simulink library "Lib_Solve_PWStateSpace_TMATS"  (R2015a)
settings: Solver=ode45  StartTime=0.0  StopTime=10.0  RelTol=1e-3
undefined symbols (not defined in the file): Atbl, Btbl, Ctbl, Dtbl, LinSys, Uo, Xo, Yo
Description:
  | Thomas Modules
settings Model: Creator=jwchapm2  LastModifiedBy=jwchapm2
settings OptimizationCC: ExpressionDepthLimit=2147483647
settings DebuggingCC: UnderspecifiedInitializationDetection=Classic  MergeDetectMultiDrivingBlocksExec=none  SolverPrmCheckMsg=warning  StateNameClashWarn=warning

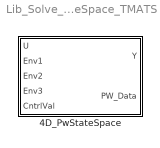
== system Lib_Solve_PWStateSpace_TMATS ==
  4D_PwStateSpace : Subsystem  mask(T-MATS: 4D Piecewise State Space Model Library Block){UisCntrl_M=off, NumEnv_M=three, XIC_M=[1 1], BN_M=double(gcb), ManDefLM_M=off, Env1_M=[0 0], Env2_M=[0 0], Env3_M=[0 0], CSVec_M=[0 0], Xsz_M=2, Ysz_M=3, Atbl_M=Atbl, Btbl_M=Btbl, Ctbl_M=Ctbl, Dtbl_M=Dtbl, Xo_M=Xo, Uo_M=Uo, Yo_M=Yo, SortEn_M=on, PLM_M=LinSys}
      mask prompts: UisCntrl_M "UisCntrl_M - Check if U is the control variable"; NumEnv_M "NumEnv_M - Number of Environmental variables"; XIC_M "XIC_M - X initial condition"; BN_M "BN_M - block name"; ManDefLM_M "ManDefLM_M - Manually define state-space model"; Env1_M "Env1_M - Environmental Vector 1 (m)"; Env2_M "Env2_M - Environmental Vector 2 (n)"; Env3_M "Env3_M - Environmental Vector 3 (p)"; CSVec_M "CSVec_M - Control Variable Vector (q)"; Xsz_M "Xnm_M - Number of states"; Ysz_M "Ynm_M - Number of outputs"; Atbl_M "Atbl_M - A matrix Array (mxnxpxqx(Xnm_M^2))"; Btbl_M "Btbl_M - B matrix Array (mxnxpxqx(Xnm_M))"; Ctbl_M "Ctbl_M - C matrix Array (mxnxpxqx(Xnm_M*Ynm_M))"; Dtbl_M "Dtbl_M - D matrix Array (mxnxpxqx(Ynm_M))"; Xo_M "Xo_M - X trim points (mxnxpxqx(Xnm_M))"; Uo_M "Uo_M - U trim points (mxnxpxq)"; Yo_M "Yo_M - Y trim points (mxnxpxqx(Ynm_M))"; SortEn_M "SortEn_M - Sort PW state-space model variables"; PLM_M "PLM_M - Piewise linear model structure name"
      mask help:
      | This block represents a 4D state-space model.
      |
      | This model will be of the form:
      | (xdot - xdot_0) = A*(x - x0) + B*(u - u0)
      | (y - y0) = C*(x - x0) + D*(u - u0)
      |
      | Where x is the system state, u is the system input (assumed to be 1x1), and y is the plant output.
      | 0 values are the trim point values.
      |
      | The 4 dimensions are represented as up to 3 "Environmental" parameters and 1 control parameter that may or may not be u. Note, if NumEnv_M is set to a value less than 3, tables must still be defined as 4D and unused Env values will be set to 0.
      mask init:
      | if NumEnv_M == 2
      |     if strcmp(get_param([BN_M '/Env2'],'BlockType'),'Constant')
      |         MSK_ReplaceBlock_TMATS([BN_M '/Env2'],'built-in/Inport');
      |     end
      |     if strcmp(get_param([BN_M '/Env3'],'BlockType'),'Inport')
      |         MSK_ReplaceBlock_TMATS([BN_M '/Env3'],'built-in/Constant');
      |         set_param([BN_M '/Env3'],'Value','[0]');
      |     end
      |     set_param([BN_M '/Env2'],'Port',num2str(3));
      | elseif NumEnv_M == 3
      |     if strcmp(get_param([BN_M '/Env2'],'BlockType'),'Constant')
      |         MSK_ReplaceBlock_TMATS([BN_M '/Env2'],'built-in/Inport');
      |     end
      |     set_param([BN_M '/Env2'],'Port',num2str(3));
      |     if strcmp(get_param([BN_M '/Env3'],'BlockType'),'Constant')
      |         MSK_ReplaceBlock_TMATS([BN_M '/Env3'],'built-in/Inport');
      |     end
      |     set_param([BN_M '/Env3'],'Port',num2str(4));
      | else
      |     if strcmp(get_param([BN_M '/Env2'],'BlockType'),'Inport')
      |         MSK_ReplaceBlock_TMATS([BN_M '/Env2'],'built-in/Constant');
      |         set_param([BN_M '/Env2'],'Value','[0]');
      |     end
      |     if strcmp(get_param([BN_M '/Env3'],'BlockType'),'Inport')
      |         MSK_ReplaceBlock_TMATS([BN_M '/Env3'],'built-in/Constant');
      |         set_param([BN_M '/Env3'],'Value','[0]');
      |     end
      | end
      | 
      | if UisCntrl_M == 0
      |     if strcmp(get_param([BN_M '/CntrlVal'],'BlockType'),'Constant')
      |         MSK_ReplaceBlock_TMATS([BN_M '/CntrlVal'],'built-in/Inport');
      |     end
      |     if NumEnv_M == 2
      |         set_param([BN_M '/CntrlVal'],'Port',num2str(4));
      |     elseif NumEnv_M == 3
      |         set_param([BN_M '/CntrlVal'],'Port',num2str(5));
      |     else
      |         set_param([BN_M '/CntrlVal'],'Port',num2str(3));
      |     end
      | elseif UisCntrl_M == 1
      |     if strcmp(get_param([BN_M '/CntrlVal'],'BlockType'),'Inport')
      |         MSK_ReplaceBlock_TMATS([BN_M '/CntrlVal'],'built-in/Constant');
      |         set_param([BN_M '/CntrlVal'],'Value','[0]');
      |     end
      | end
      | 
      | if ManDefLM_M
      |     %Manually define Linear model structure
      |     %Input axis vectors 4d
      |     PLM_M.EVec{1} = Env1_M;
      |     PLM_M.EVec{2} = Env2_M;
      |     PLM_M.EVec{3} = Env3_M;
      |     PLM_M.CSVec  = CSVec_M;
      |     %matrix sizes
      |     PLM_M.Asize = [Xsz_M Xsz_M];
      |     PLM_M.Bsize = [Xsz_M 1];
      |     PLM_M.Csize = [Ysz_M Xsz_M];
      |     PLM_M.Dsize = [Ysz_M 1];
      |     PLM_M.Xosize = [Xsz_M 1];
      |     PLM_M.Yosize = [Ysz_M 1];
      |     PLM_M.Uosize = 1;
      |     
      |     %define 5d tables (4d lookup, extra d relates different matrix
      |     %elements, ie. A11, A12,A21, A22.
      |     PLM_M.AtblFE = Atbl_M;
      |     PLM_M.BtblFE = Btbl_M;
      |     PLM_M.CtblFE = Ctbl_M;
      |     PLM_M.DtblFE = Dtbl_M;
      |     
      |     PLM_M.XoFE = Xo_M;
      |     PLM_M.UoFE = Uo_M;
      |     PLM_M.YoFE = Yo_M;
      | else
      |     % use structure linear system input... sort if necessary
      |     LS = PLM_M;
      |     
      |     if isfield(LS,'TblGen')
      |         if LS.TblGen == true;
      |             SortData = false;
      |         else
      |             SortData = true;
      |         end
      |     elseif all(isfield(LS,{'ABCD','EnvVec','X','U','Y','CntrlSlew'}))
      |         SortData = true;
      |     else
      |         SortData = false;
      |         sprintf(strcat('Warning in block: ',BN_M, ' Can not Sort out Linear system data due to improper PLM_M structure definition'))
      |     end
      |     
      |     if SortData == true && SortEn_M
      |         LS = TMATS_PWSort(LS);
      |         assignin('base','LinSys_Sorted',LS);
      |         PLM_M = LS;
      |     end
      | end
      mask Help: web(which('Solver_TMATS_PWSS.html'),'-helpbrowser')
      mask TypeOptions NumEnv_M: one | two | three
      mask Callback ManDefLM_M:
      | MSK_SEC_Enables_TMATS('ManDefLM_M',[6:18],'en')
      | MSK_SEC_Enables_TMATS('ManDefLM_M',[20],'dis')
      mask DialogControl Control2 Prompt: This tab is used when the state space model is defined using a structure.  (see block help)
      mask DialogControl Control2_copy Prompt: If this structure was generated using the T-MATS PW linear model generator, SortEn_M should be checked.

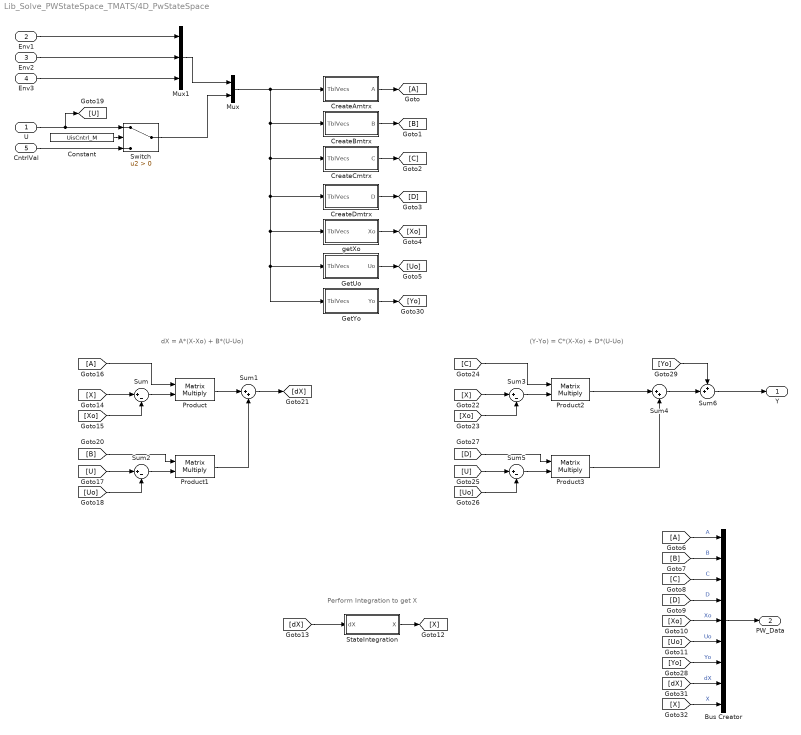
== system Lib_Solve_PWStateSpace_TMATS/4D_PwStateSpace ==
  note: dX = A*(X-Xo) + B*(U-Uo)
  note: Perform Integration to get X
  note: (Y-Yo) = C*(X-Xo) + D*(U-Uo)
  U : Inport
  Env1 : Inport  Port=2
  Env2 : Inport  Port=3
  Env3 : Inport  Port=4
  CntrlVal : Inport  Port=5
  Bus Creator : BusCreator  Inputs=9
  Constant : Constant  Value=UisCntrl_M
  CreateAmtrx : Subsystem
  CreateBmtrx : Subsystem
  CreateCmtrx : Subsystem
  CreateDmtrx : Subsystem
  GetUo : Subsystem
  GetYo : Subsystem
  Mux : Mux  Inputs=[3 1]
  Mux1 : Mux  Inputs=3
  Product{,1..3} (4 alike) : Product  Multiplication=Matrix(*)
  StateIntegration : Subsystem
  Sum{,2..3,5} (4 alike) : Sum  Inputs=|+-
  Sum1 : Sum  Inputs=|++
  Sum4 : Sum  Inputs=|++
  Sum6 : Sum  Inputs=++|
  Switch : Switch  Criteria=u2 > Threshold
  getXo : Subsystem
  Y : Outport
  PW_Data : Outport  Port=2
  wires:
  [X] -> Bus Creator/9  "X"
  [dX] -> Bus Creator/8  "dX"
  GetYo/1(Yo) -> [Yo]
  [Xo] -> Bus Creator/5  "Xo"
  [D] -> Bus Creator/4  "D"
  [C] -> Bus Creator/3  "C"
  [Uo] -> Bus Creator/6  "Uo"
  [B] -> Bus Creator/2  "B"
  [A] -> Bus Creator/1  "A"
  GetUo/1(Uo) -> [Uo]
  getXo/1(Xo) -> [Xo]
  U/1 -> [U], Switch/1
  CreateBmtrx/1(B) -> [B]
  CreateCmtrx/1(C) -> [C]
  CreateDmtrx/1(D) -> [D]
  Bus Creator/1 -> PW_Data/1
  [X] -> Sum/1
  [Xo] -> Sum/2
  Sum/1 -> Product/2
  [A] -> Product/1
  Product/1 -> Sum1/1
  [U] -> Sum2/1
  [Uo] -> Sum2/2
  Sum2/1 -> Product1/2
  [B] -> Product1/1
  Product1/1 -> Sum1/2
  Sum1/1 -> [dX]
  [X] -> Sum3/1
  [Xo] -> Sum3/2
  Sum3/1 -> Product2/2
  [C] -> Product2/1
  Product2/1 -> Sum4/1
  [U] -> Sum5/1
  [Uo] -> Sum5/2
  Sum5/1 -> Product3/2
  [D] -> Product3/1
  Product3/1 -> Sum4/2
  Sum6/1 -> Y/1
  Sum4/1 -> Sum6/2
  [Yo] -> Sum6/1
  [Yo] -> Bus Creator/7  "Yo"
  Env1/1 -> Mux1/1
  Constant/1 -> Switch/2
  CntrlVal/1 -> Switch/3
  CreateAmtrx/1(A) -> [A]
  Mux1/1 -> Mux/1
  Switch/1 -> Mux/2
  Mux/1 -> CreateBmtrx/1(TblVecs), CreateCmtrx/1(TblVecs), CreateDmtrx/1(TblVecs), getXo/1(TblVecs), GetUo/1(TblVecs), GetYo/1(TblVecs), CreateAmtrx/1(TblVecs)
  [dX] -> StateIntegration/1(dX)
  StateIntegration/1(X) -> [X]
  Env2/1 -> Mux1/2
  Env3/1 -> Mux1/3

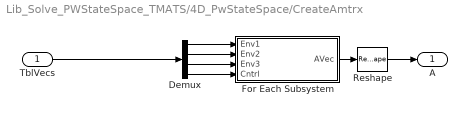
== system Lib_Solve_PWStateSpace_TMATS/4D_PwStateSpace/CreateAmtrx ==
  TblVecs : Inport
  Demux : Demux
  For Each Subsystem : Subsystem  TreatAsAtomicUnit=on  mask{Table=PLM_M.AtblFE}
  Reshape : Reshape  OutputDimensionality=Customize  OutputDimensions=PLM_M.Asize
  A : Outport
  wires:
  TblVecs/1 -> Demux/1
  Demux/2 -> For Each Subsystem/2(Env2)
  Reshape/1 -> A/1
  For Each Subsystem/1(AVec) -> Reshape/1
  Demux/3 -> For Each Subsystem/3(Env3)
  Demux/1 -> For Each Subsystem/1(Env1)
  Demux/4 -> For Each Subsystem/4(Cntrl)

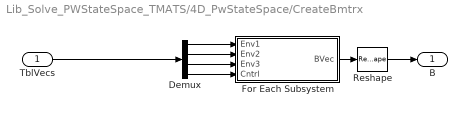
== system Lib_Solve_PWStateSpace_TMATS/4D_PwStateSpace/CreateBmtrx ==
  TblVecs : Inport
  Demux : Demux
  For Each Subsystem : Subsystem  TreatAsAtomicUnit=on  mask{Table=PLM_M.BtblFE}
  Reshape : Reshape  OutputDimensionality=Customize  OutputDimensions=PLM_M.Bsize
  B : Outport
  wires:
  Demux/4 -> For Each Subsystem/4(Cntrl)
  Demux/1 -> For Each Subsystem/1(Env1)
  Demux/3 -> For Each Subsystem/3(Env3)
  For Each Subsystem/1(BVec) -> Reshape/1
  Reshape/1 -> B/1
  Demux/2 -> For Each Subsystem/2(Env2)
  TblVecs/1 -> Demux/1

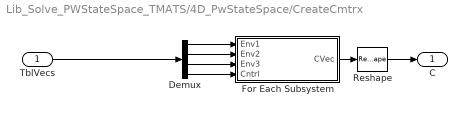
== system Lib_Solve_PWStateSpace_TMATS/4D_PwStateSpace/CreateCmtrx ==
  TblVecs : Inport
  Demux : Demux
  For Each Subsystem : Subsystem  TreatAsAtomicUnit=on  mask{Table=PLM_M.CtblFE}
  Reshape : Reshape  OutputDimensionality=Customize  OutputDimensions=PLM_M.Csize
  C : Outport
  wires:
  TblVecs/1 -> Demux/1
  Demux/2 -> For Each Subsystem/2(Env2)
  Reshape/1 -> C/1
  For Each Subsystem/1(CVec) -> Reshape/1
  Demux/3 -> For Each Subsystem/3(Env3)
  Demux/1 -> For Each Subsystem/1(Env1)
  Demux/4 -> For Each Subsystem/4(Cntrl)

== system Lib_Solve_PWStateSpace_TMATS/4D_PwStateSpace/CreateDmtrx ==
  TblVecs : Inport
  Demux : Demux
  For Each Subsystem : Subsystem  TreatAsAtomicUnit=on  mask{Table=PLM_M.DtblFE}
  Reshape : Reshape  OutputDimensionality=Customize  OutputDimensions=PLM_M.Dsize
  D : Outport
  wires:
  Demux/4 -> For Each Subsystem/4(Cntrl)
  Demux/1 -> For Each Subsystem/1(Env1)
  Demux/3 -> For Each Subsystem/3(Env3)
  For Each Subsystem/1(DVec) -> Reshape/1
  Reshape/1 -> D/1
  Demux/2 -> For Each Subsystem/2(Env2)
  TblVecs/1 -> Demux/1

== system Lib_Solve_PWStateSpace_TMATS/4D_PwStateSpace/GetUo ==
  TblVecs : Inport
  Demux : Demux
  Table lookup : Subsystem  TreatAsAtomicUnit=on  mask{Table=PLM_M.UoFE}
  Uo : Outport
  wires:
  Demux/4 -> Table lookup/4(Cntrl)
  Demux/1 -> Table lookup/1(Env1)
  Demux/3 -> Table lookup/3(Env3)
  Table lookup/1(UoVec) -> Uo/1
  Demux/2 -> Table lookup/2(Env2)
  TblVecs/1 -> Demux/1

== system Lib_Solve_PWStateSpace_TMATS/4D_PwStateSpace/GetYo ==
  TblVecs : Inport
  Demux : Demux
  For Each Subsystem : Subsystem  TreatAsAtomicUnit=on  mask{Table=PLM_M.YoFE}
  Reshape : Reshape  OutputDimensionality=Customize  OutputDimensions=PLM_M.Yosize
  Yo : Outport
  wires:
  Demux/4 -> For Each Subsystem/4(Cntrl)
  Demux/1 -> For Each Subsystem/1(Env1)
  Demux/3 -> For Each Subsystem/3(Env3)
  For Each Subsystem/1(YoVec) -> Reshape/1
  Reshape/1 -> Yo/1
  Demux/2 -> For Each Subsystem/2(Env2)
  TblVecs/1 -> Demux/1

== system Lib_Solve_PWStateSpace_TMATS/4D_PwStateSpace/StateIntegration ==
  dX : Inport  PortDimensions=length(XIC_M)
  Integrator : Integrator  InitialCondition=XIC_M
  X : Outport  PortDimensions=length(XIC_M)
  wires:
  Integrator/1 -> X/1
  dX/1 -> Integrator/1

== system Lib_Solve_PWStateSpace_TMATS/4D_PwStateSpace/getXo ==
  TblVecs : Inport
  Demux : Demux
  For Each Subsystem : Subsystem  TreatAsAtomicUnit=on  mask{Table=PLM_M.XoFE}
  Reshape : Reshape  OutputDimensionality=Customize  OutputDimensions=PLM_M.Xosize
  Xo : Outport
  wires:
  TblVecs/1 -> Demux/1
  Demux/2 -> For Each Subsystem/2(Env2)
  Reshape/1 -> Xo/1
  For Each Subsystem/1(XoVec) -> Reshape/1
  Demux/3 -> For Each Subsystem/3(Env3)
  Demux/1 -> For Each Subsystem/1(Env1)
  Demux/4 -> For Each Subsystem/4(Cntrl)

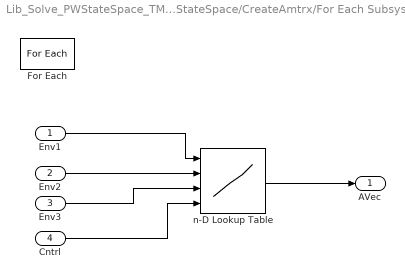
== system Lib_Solve_PWStateSpace_TMATS/4D_PwStateSpace/CreateAmtrx/For Each Subsystem ==
  Env1 : Inport  Partition=off
  Env2 : Inport  Port=2  Partition=off
  Env3 : Inport  Port=3  Partition=off
  Cntrl : Inport  Port=4  Partition=off
  For Each : ForEach  DisableCoverage=on  IterateSubsysMaskParameter=on  SubsysMaskParameterIterationDimension=5  IndexMode=One-based
  n-D Lookup Table : Lookup_n-D  NumberOfTableDimensions=4  BreakpointsForDimension1=PLM_M.EVec{1}  BreakpointsForDimension2=PLM_M.EVec{2}  BreakpointsForDimension3=PLM_M.EVec{3}  BreakpointsForDimension4=PLM_M.CSVec  Table=Table  InternalRulePriority=Speed  RndMeth=Simplest  InputSameDT=on
  AVec : Outport  ConcatenationDimension=1
  wires:
  n-D Lookup Table/1 -> AVec/1
  Cntrl/1 -> n-D Lookup Table/4
  Env3/1 -> n-D Lookup Table/3
  Env2/1 -> n-D Lookup Table/2
  Env1/1 -> n-D Lookup Table/1

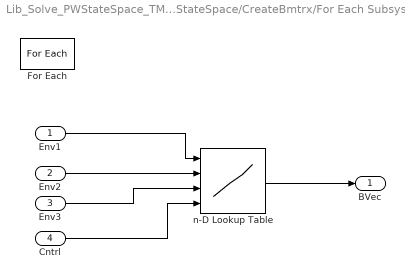
== system Lib_Solve_PWStateSpace_TMATS/4D_PwStateSpace/CreateBmtrx/For Each Subsystem ==
  Env1 : Inport  Partition=off
  Env2 : Inport  Port=2  Partition=off
  Env3 : Inport  Port=3  Partition=off
  Cntrl : Inport  Port=4  Partition=off
  For Each : ForEach  DisableCoverage=on  IterateSubsysMaskParameter=on  SubsysMaskParameterIterationDimension=5  IndexMode=One-based
  n-D Lookup Table : Lookup_n-D  NumberOfTableDimensions=4  BreakpointsForDimension1=PLM_M.EVec{1}  BreakpointsForDimension2=PLM_M.EVec{2}  BreakpointsForDimension3=PLM_M.EVec{3}  BreakpointsForDimension4=PLM_M.CSVec  Table=Table  InternalRulePriority=Speed  RndMeth=Simplest  InputSameDT=on
  BVec : Outport  ConcatenationDimension=1
  wires:
  Env1/1 -> n-D Lookup Table/1
  Env2/1 -> n-D Lookup Table/2
  Env3/1 -> n-D Lookup Table/3
  Cntrl/1 -> n-D Lookup Table/4
  n-D Lookup Table/1 -> BVec/1

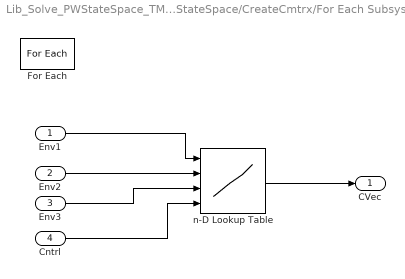
== system Lib_Solve_PWStateSpace_TMATS/4D_PwStateSpace/CreateCmtrx/For Each Subsystem ==
  Env1 : Inport  Partition=off
  Env2 : Inport  Port=2  Partition=off
  Env3 : Inport  Port=3  Partition=off
  Cntrl : Inport  Port=4  Partition=off
  For Each : ForEach  DisableCoverage=on  IterateSubsysMaskParameter=on  SubsysMaskParameterIterationDimension=5  IndexMode=One-based
  n-D Lookup Table : Lookup_n-D  NumberOfTableDimensions=4  BreakpointsForDimension1=PLM_M.EVec{1}  BreakpointsForDimension2=PLM_M.EVec{2}  BreakpointsForDimension3=PLM_M.EVec{3}  BreakpointsForDimension4=PLM_M.CSVec  Table=Table  InternalRulePriority=Speed  RndMeth=Simplest  InputSameDT=on
  CVec : Outport  ConcatenationDimension=1
  wires:
  n-D Lookup Table/1 -> CVec/1
  Cntrl/1 -> n-D Lookup Table/4
  Env3/1 -> n-D Lookup Table/3
  Env2/1 -> n-D Lookup Table/2
  Env1/1 -> n-D Lookup Table/1

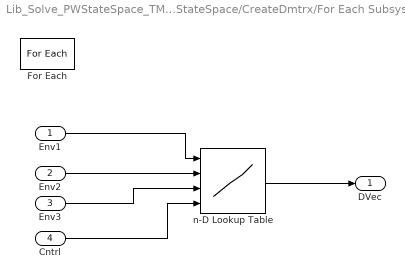
== system Lib_Solve_PWStateSpace_TMATS/4D_PwStateSpace/CreateDmtrx/For Each Subsystem ==
  Env1 : Inport  Partition=off
  Env2 : Inport  Port=2  Partition=off
  Env3 : Inport  Port=3  Partition=off
  Cntrl : Inport  Port=4  Partition=off
  For Each : ForEach  DisableCoverage=on  IterateSubsysMaskParameter=on  SubsysMaskParameterIterationDimension=5  IndexMode=One-based
  n-D Lookup Table : Lookup_n-D  NumberOfTableDimensions=4  BreakpointsForDimension1=PLM_M.EVec{1}  BreakpointsForDimension2=PLM_M.EVec{2}  BreakpointsForDimension3=PLM_M.EVec{3}  BreakpointsForDimension4=PLM_M.CSVec  Table=Table  InternalRulePriority=Speed  RndMeth=Simplest  InputSameDT=on
  DVec : Outport  ConcatenationDimension=1
  wires:
  Env1/1 -> n-D Lookup Table/1
  Env2/1 -> n-D Lookup Table/2
  Env3/1 -> n-D Lookup Table/3
  Cntrl/1 -> n-D Lookup Table/4
  n-D Lookup Table/1 -> DVec/1

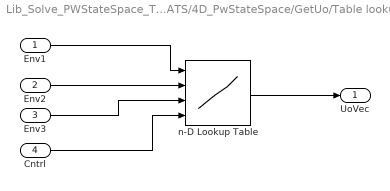
== system Lib_Solve_PWStateSpace_TMATS/4D_PwStateSpace/GetUo/Table lookup ==
  Env1 : Inport
  Env2 : Inport  Port=2
  Env3 : Inport  Port=3
  Cntrl : Inport  Port=4
  n-D Lookup Table : Lookup_n-D  NumberOfTableDimensions=4  BreakpointsForDimension1=PLM_M.EVec{1}  BreakpointsForDimension2=PLM_M.EVec{2}  BreakpointsForDimension3=PLM_M.EVec{3}  BreakpointsForDimension4=PLM_M.CSVec  Table=Table  InternalRulePriority=Speed  RndMeth=Simplest  InputSameDT=on
  UoVec : Outport
  wires:
  Env1/1 -> n-D Lookup Table/1
  Env2/1 -> n-D Lookup Table/2
  Env3/1 -> n-D Lookup Table/3
  Cntrl/1 -> n-D Lookup Table/4
  n-D Lookup Table/1 -> UoVec/1

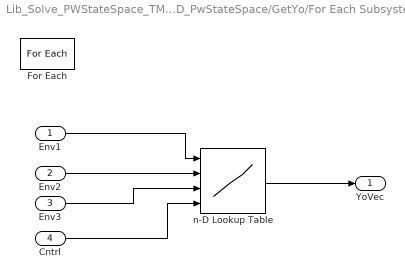
== system Lib_Solve_PWStateSpace_TMATS/4D_PwStateSpace/GetYo/For Each Subsystem ==
  Env1 : Inport  Partition=off
  Env2 : Inport  Port=2  Partition=off
  Env3 : Inport  Port=3  Partition=off
  Cntrl : Inport  Port=4  Partition=off
  For Each : ForEach  DisableCoverage=on  IterateSubsysMaskParameter=on  SubsysMaskParameterIterationDimension=5  IndexMode=One-based
  n-D Lookup Table : Lookup_n-D  NumberOfTableDimensions=4  BreakpointsForDimension1=PLM_M.EVec{1}  BreakpointsForDimension2=PLM_M.EVec{2}  BreakpointsForDimension3=PLM_M.EVec{3}  BreakpointsForDimension4=PLM_M.CSVec  Table=Table  InternalRulePriority=Speed  RndMeth=Simplest  InputSameDT=on
  YoVec : Outport  ConcatenationDimension=1
  wires:
  Env1/1 -> n-D Lookup Table/1
  Env2/1 -> n-D Lookup Table/2
  Env3/1 -> n-D Lookup Table/3
  Cntrl/1 -> n-D Lookup Table/4
  n-D Lookup Table/1 -> YoVec/1

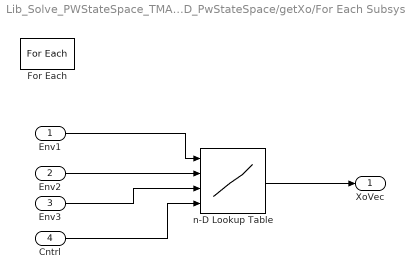
== system Lib_Solve_PWStateSpace_TMATS/4D_PwStateSpace/getXo/For Each Subsystem ==
  Env1 : Inport  Partition=off
  Env2 : Inport  Port=2  Partition=off
  Env3 : Inport  Port=3  Partition=off
  Cntrl : Inport  Port=4  Partition=off
  For Each : ForEach  DisableCoverage=on  IterateSubsysMaskParameter=on  SubsysMaskParameterIterationDimension=5  IndexMode=One-based
  n-D Lookup Table : Lookup_n-D  NumberOfTableDimensions=4  BreakpointsForDimension1=PLM_M.EVec{1}  BreakpointsForDimension2=PLM_M.EVec{2}  BreakpointsForDimension3=PLM_M.EVec{3}  BreakpointsForDimension4=PLM_M.CSVec  Table=Table  InternalRulePriority=Speed  RndMeth=Simplest  InputSameDT=on
  XoVec : Outport  ConcatenationDimension=1
  wires:
  n-D Lookup Table/1 -> XoVec/1
  Cntrl/1 -> n-D Lookup Table/4
  Env3/1 -> n-D Lookup Table/3
  Env2/1 -> n-D Lookup Table/2
  Env1/1 -> n-D Lookup Table/1
